simulink model "simu"  (R2012b)
settings: Solver=ode45  StartTime=0.0  StopTime=0.01  RelTol=1e-3
undefined symbols (not defined in the file): br, cr, Jr, kr
settings Model: Creator=Felipe  LastModifiedBy=Felipe

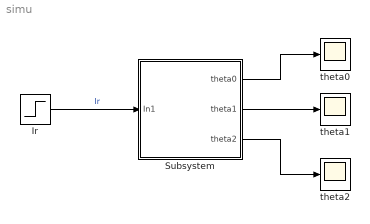
== system simu ==
  Ir : Step  Time=5  Before=2  After=5  SampleTime=0
  Subsystem : Subsystem
  theta0 : Scope
      settings: YMin=1.55e-07  YMax=2.35e-07
  theta1 : Scope
      settings: YMin=-6e-06  YMax=1e-05
  theta2 : Scope
      settings: SaveName=ScopeData2
  wires:
  Ir/1 -> Subsystem/1(In1)  "Ir"
  Subsystem/1(theta0) -> theta0/1
  Subsystem/2(theta1) -> theta1/1
  Subsystem/3(theta2) -> theta2/1

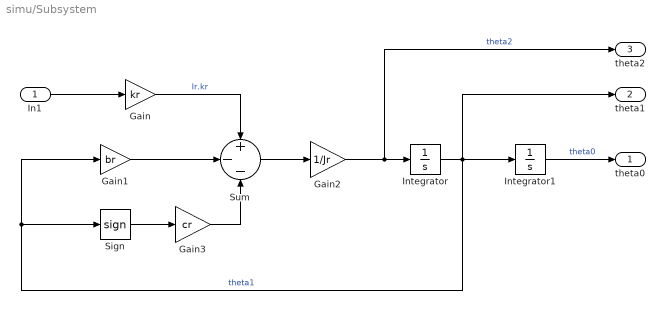
== system simu/Subsystem ==
  In1 : Inport
  Gain : Gain  Gain=kr
  Gain1 : Gain  Gain=br
  Gain2 : Gain  Gain=1/Jr
  Gain3 : Gain  Gain=cr
  Integrator : Integrator
  Integrator1 : Integrator
  Sign : Signum  ZeroCross=off
  Sum : Sum  Inputs=+--
  theta0 : Outport
  theta1 : Outport  Port=2
  theta2 : Outport  Port=3
  wires:
  Integrator/1 -> theta1/1, Sign/1, Gain1/1, Integrator1/1  "theta1"
  Integrator1/1 -> theta0/1  "theta0"
  Gain2/1 -> theta2/1, Integrator/1  "theta2"
  Gain/1 -> Sum/1  "Ir.kr"
  Sum/1 -> Gain2/1
  Gain1/1 -> Sum/2
  In1/1 -> Gain/1
  Gain3/1 -> Sum/3
  Sign/1 -> Gain3/1
